simulink model "autopilot"  (R2016a)
settings: Solver=VariableStepAuto  StartTime=0.0  StopTime=10  RelTol=1e-3
values from neighbouring files (symbols this model uses):
  A = [-0.727 345.2118852 0 ... (first row only)    [linear_model.m]
  B = [-20.7 ; -23.5 ; 0]    [linear_model.m]
  K = [0.0031   -0.7217   -7.7460]    [state_dot_fn2.m]
  Nbar = K(3)    [linear_model.m]
settings Model: Creator=M  LastModifiedBy=M

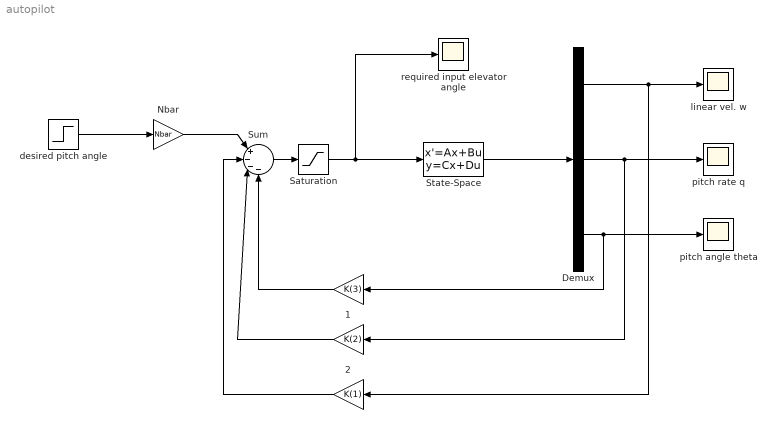
== system autopilot ==
  " " : Gain  Gain=K(3)
  " 1" : Gain  Gain=K(2)
  " 2" : Gain  Gain=K(1)
  Demux : Demux  Outputs=3
  Nbar : Gain  Gain=Nbar
  Saturation : Saturate  UpperLimit=.5  LowerLimit=-.5
  State-Space : StateSpace  A=A  B=B  C=eye(3)  D=[0;0;0]  X0=0
  Sum : Sum  Inputs=|+---
  desired pitch angle : Step  Time=0  After=0.3  SampleTime=0.1
  linear vel. w : Scope
  pitch angle theta : Scope
  pitch rate q : Scope
  required input elevator angle : Scope
  wires:
  Sum/1 -> Saturation/1
  desired pitch angle/1 -> Nbar/1
  Saturation/1 -> required input elevator angle/1, State-Space/1
  State-Space/1 -> Demux/1
  " "/1 -> Sum/4
  Nbar/1 -> Sum/1
  Demux/2 -> pitch rate q/1, " 1"/1
  Demux/3 -> " "/1, pitch angle theta/1
  " 1"/1 -> Sum/3
  " 2"/1 -> Sum/2
  Demux/1 -> linear vel. w/1, " 2"/1
